simulink model "PassengerCar"  (R2019b)
settings: Solver=ode1  StartTime=0  StopTime=25  FixedStep=1.0000000000000000e-003  RelTol=1e-3
InitFcn:
  | sampleTime = str2double(get_param(bdroot, 'FixedStep'));
undefined symbols (not defined in the file or in its folder): AccPedalPos, BrakePedalPos, BrakeSwitch, DiscIntNeverNeededParam, DYNA4, EngSpd, IgnitionSwitch, InitialGear, InitialSpeed, IntendedEngTrq, LeftIndicator, MainBrakePress, MaxGear, MDL, MinGear, RefAcc, RefLane, RefLatPos, RefPath, RefPathCurv, RefSpd, RefSpdPreview, RefSpdRetrospect, RightIndicator, SteeringWheelAng, SteeringWheelTrq, UserDefinedRefValue, vm_const
libraries: UtilitiesLibrary x31, simulink x18, WheelSystemModules x13, LongitudinalControllerModules x13, LateralControllerModules x7, AnimationBusselectorModules x5, EnvironmentModules x5, BasicEngineControlModules x5, MiscellaneousControlModules x5, Animation3Modules x4, AuxiliariesModules x4, TireModules x4
(part 25 of 39)

== system PassengerCar/Vehicle/WheelSystem/RearLeftWheelSystem/WheelOutput ==
  DriveBrakeTrq_wrt_WheelRotAxis(VehSys)[Nm]___UNIQUE_1 : Inport  Description=|  PortDimensions=[3]
      | <name>DriveBrakeTrq_wrt_WheelRotAxis(VehSys)[Nm]</name>
      | <comment></comment>
  RotSpd[rad/s]___UNIQUE_1 : Inport  Description=|  Port=2  PortDimensions=[1]
      | <name>RotSpd[rad/s]</name>
      | <comment></comment>
  RotAcc[rad/s**2]___UNIQUE_1 : Inport  Description=|  Port=3  PortDimensions=[1]
      | <name>RotAcc[rad/s**2]</name>
      | <comment></comment>
  BlockingState[0;1]___UNIQUE_1 : Inport  Description=|  Port=4  PortDimensions=[1]
      | <name>BlockingState[0;1]</name>
      | <comment></comment>
  RotAng[rad]___UNIQUE_1 : Inport  Description=|  Port=5  PortDimensions=[1]
      | <name>RotAng[rad]</name>
      | <comment></comment>
  BrakeTrqPressRatio[m**3]___UNIQUE_1 : Inport  Description=|  Port=6  PortDimensions=[1]
      | <name>BrakeTrqPressRatio[m**3]</name>
      | <comment></comment>
  RotAxisInrt[kg*m**2]___UNIQUE_1 : Inport  Description=|  Port=7  PortDimensions=[1]
      | <name>RotAxisInrt[kg*m**2]</name>
      | <comment></comment>
  TotalResistanceTorque[Nm]___UNIQUE_1 : Inport  Description=|  Port=8  PortDimensions=[1]
      | <name>TotalResistanceTorque[Nm]</name>
      | <comment></comment>
  KinematicWheelActiveFlag[0;1]___UNIQUE_1 : Inport  Description=|  Port=9  PortDimensions=[1]
      | <name>KinematicWheelActiveFlag[0;1]</name>
      | <comment></comment>
  VehBodyReplacementInrt[kg*m**2]___UNIQUE_1 : Inport  Description=|  Port=10  PortDimensions=[1]
      | <name>VehBodyReplacementInrt[kg*m**2]</name>
      | <comment></comment>
  __TDD__Wheel.BlockingState[0;1] : Demux  Outputs=[1]
  __TDD__Wheel.BrakeTrqPressRatio[m**3] : Demux  Outputs=[1]
  __TDD__Wheel.DriveBrakeTrq_wrt_WheelRotAxis(VehSys)[Nm] : Demux  Outputs=[3]
  __TDD__Wheel.KinematicWheelActiveFlag[0;1] : Demux  Outputs=[1]
  __TDD__Wheel.RotAcc[rad/s**2] : Demux  Outputs=[1]
  __TDD__Wheel.RotAng[rad] : Demux  Outputs=[1]
  __TDD__Wheel.RotAxisInrt[kg*m**2] : Demux  Outputs=[1]
  __TDD__Wheel.RotSpd[rad/s] : Demux  Outputs=[1]
  __TDD__Wheel.TotalResistanceTorque[Nm] : Demux  Outputs=[1]
  __TDD__Wheel.VehBodyReplacementInrt[kg*m**2] : Demux  Outputs=[1]
  __TDO__Wheel : BusCreator  Inputs=10
  Wheel___UNIQUE_1 : Outport  Description=|  PortDimensions=[12]  VectorParamsAs1DForOutWhenUnconnected=off
      | <name>DriveBrakeTrq_wrt_WheelRotAxis(VehSys)[Nm]</name>
      | <comment></comment>
  wires:
  DriveBrakeTrq_wrt_WheelRotAxis(VehSys)[Nm]___UNIQUE_1/1 -> __TDD__Wheel.DriveBrakeTrq_wrt_WheelRotAxis(VehSys)[Nm]/1
  __TDD__Wheel.DriveBrakeTrq_wrt_WheelRotAxis(VehSys)[Nm]/1 -> __TDO__Wheel/1  "DriveBrakeTrq_wrt_WheelRotAxis(VehSys)[Nm]"
  RotSpd[rad/s]___UNIQUE_1/1 -> __TDD__Wheel.RotSpd[rad/s]/1
  __TDD__Wheel.RotSpd[rad/s]/1 -> __TDO__Wheel/2  "RotSpd[rad/s]"
  RotAcc[rad/s**2]___UNIQUE_1/1 -> __TDD__Wheel.RotAcc[rad/s**2]/1
  __TDD__Wheel.RotAcc[rad/s**2]/1 -> __TDO__Wheel/3  "RotAcc[rad/s**2]"
  BlockingState[0;1]___UNIQUE_1/1 -> __TDD__Wheel.BlockingState[0;1]/1
  __TDD__Wheel.BlockingState[0;1]/1 -> __TDO__Wheel/4  "BlockingState[0;1]"
  RotAng[rad]___UNIQUE_1/1 -> __TDD__Wheel.RotAng[rad]/1
  __TDD__Wheel.RotAng[rad]/1 -> __TDO__Wheel/5  "RotAng[rad]"
  BrakeTrqPressRatio[m**3]___UNIQUE_1/1 -> __TDD__Wheel.BrakeTrqPressRatio[m**3]/1
  __TDD__Wheel.BrakeTrqPressRatio[m**3]/1 -> __TDO__Wheel/6  "BrakeTrqPressRatio[m**3]"
  RotAxisInrt[kg*m**2]___UNIQUE_1/1 -> __TDD__Wheel.RotAxisInrt[kg*m**2]/1
  __TDD__Wheel.RotAxisInrt[kg*m**2]/1 -> __TDO__Wheel/7  "RotAxisInrt[kg*m**2]"
  TotalResistanceTorque[Nm]___UNIQUE_1/1 -> __TDD__Wheel.TotalResistanceTorque[Nm]/1
  __TDD__Wheel.TotalResistanceTorque[Nm]/1 -> __TDO__Wheel/8  "TotalResistanceTorque[Nm]"
  KinematicWheelActiveFlag[0;1]___UNIQUE_1/1 -> __TDD__Wheel.KinematicWheelActiveFlag[0;1]/1
  __TDD__Wheel.KinematicWheelActiveFlag[0;1]/1 -> __TDO__Wheel/9  "KinematicWheelActiveFlag[0;1]"
  VehBodyReplacementInrt[kg*m**2]___UNIQUE_1/1 -> __TDD__Wheel.VehBodyReplacementInrt[kg*m**2]/1
  __TDD__Wheel.VehBodyReplacementInrt[kg*m**2]/1 -> __TDO__Wheel/10  "VehBodyReplacementInrt[kg*m**2]"
  __TDO__Wheel/1 -> Wheel___UNIQUE_1/1  "Wheel"

== system PassengerCar/Vehicle/WheelSystem/RearRightWheelSystem/DynaSystemInfo ==

== system PassengerCar/Vehicle/WheelSystem/RearRightWheelSystem/InnerTireOutput ==
  __SEL__Tire.ContactPointFrc(ContactSys)[N] : Selector  InputPortWidth=1  IndexOptions=Index vector (dialog)  Indices=ones(3, 1)  OutputSizes=1
  __SEL__Tire.ContactPointPos(WorldSys)[m] : Selector  InputPortWidth=1  IndexOptions=Index vector (dialog)  Indices=ones(3, 1)  OutputSizes=1
  __SEL__Tire.ContactPointPos_wrt_WheelCenter(WorldSys)[m] : Selector  InputPortWidth=1  IndexOptions=Index vector (dialog)  Indices=ones(3, 1)  OutputSizes=1
  __SEL__Tire.LatUnitVector(WorldSys)[-] : Selector  InputPortWidth=1  IndexOptions=Index vector (dialog)  Indices=ones(3, 1)  OutputSizes=1
  __SEL__Tire.LongUnitVector(WorldSys)[-] : Selector  InputPortWidth=1  IndexOptions=Index vector (dialog)  Indices=ones(3, 1)  OutputSizes=1
  __SEL__Tire.RoadNormalVector(WorldSys)[-] : Selector  InputPortWidth=1  IndexOptions=Index vector (dialog)  Indices=ones(3, 1)  OutputSizes=1
  __SEL__Tire.WheelCenterFrc(VehSys)[N] : Selector  InputPortWidth=1  IndexOptions=Index vector (dialog)  Indices=ones(3, 1)  OutputSizes=1
  __SEL__Tire.WheelCenterTrq(VehSys)[Nm] : Selector  InputPortWidth=1  IndexOptions=Index vector (dialog)  Indices=ones(3, 1)  OutputSizes=1
  __SRC__Tire.BoreSpd(ContactSys)[rad/s] : Constant  Value=0.0  OutDataTypeStr=Inherit: Inherit via back propagation
  __SRC__Tire.CamberAng(ContactSys)[rad] : Constant  Value=0.0  OutDataTypeStr=Inherit: Inherit via back propagation
  __SRC__Tire.CircumferentialTrq_wrt_WheelRotAxis[Nm] : Constant  Value=0.0  OutDataTypeStr=Inherit: Inherit via back propagation
  __SRC__Tire.ContactPointFrc(ContactSys)[N] : Constant  Value=0.0  OutDataTypeStr=Inherit: Inherit via back propagation
  __SRC__Tire.ContactPointPos(WorldSys)[m] : Constant  Value=0.0  OutDataTypeStr=Inherit: Inherit via back propagation
  __SRC__Tire.ContactPointPos_wrt_WheelCenter(WorldSys)[m] : Constant  Value=0.0  OutDataTypeStr=Inherit: Inherit via back propagation
  __SRC__Tire.CorneringStiff[N] : Constant  Value=0.0  OutDataTypeStr=Inherit: Inherit via back propagation
  __SRC__Tire.DynamicRadius[m] : Constant  Value=0.0  OutDataTypeStr=Inherit: Inherit via back propagation
  __SRC__Tire.LatDefl(ContactSys)[m] : Constant  Value=0.0  OutDataTypeStr=Inherit: Inherit via back propagation
  __SRC__Tire.LatSpd(ContactSys)[m/s] : Constant  Value=0.0  OutDataTypeStr=Inherit: Inherit via back propagation
  __SRC__Tire.LatUnitVector(WorldSys)[-] : Constant  Value=0.0  OutDataTypeStr=Inherit: Inherit via back propagation
  __SRC__Tire.LongFrcLeverArm_wrt_WheelRotAxis[m] : Constant  Value=0.0  OutDataTypeStr=Inherit: Inherit via back propagation
  __SRC__Tire.LongSpd(ContactSys)[m/s] : Constant  Value=0.0  OutDataTypeStr=Inherit: Inherit via back propagation
  __SRC__Tire.LongUnitVector(WorldSys)[-] : Constant  Value=0.0  OutDataTypeStr=Inherit: Inherit via back propagation
  __SRC__Tire.MaxRollResistTrq[Nm] : Constant  Value=0.0  OutDataTypeStr=Inherit: Inherit via back propagation
  __SRC__Tire.RimRadius[m] : Constant  Value=0.0  OutDataTypeStr=Inherit: Inherit via back propagation
  __SRC__Tire.RoadFrictionScalingCoeff[-] : Constant  Value=0.0  OutDataTypeStr=Inherit: Inherit via back propagation
  __SRC__Tire.RoadIncl(WorldSys)[-] : Constant  Value=0.0  OutDataTypeStr=Inherit: Inherit via back propagation
  __SRC__Tire.RoadNormalVector(WorldSys)[-] : Constant  Value=0.0  OutDataTypeStr=Inherit: Inherit via back propagation
  __SRC__Tire.RoadSlope(WorldSys)[-] : Constant  Value=0.0  OutDataTypeStr=Inherit: Inherit via back propagation
  __SRC__Tire.RoadType[-] : Constant  Value=0.0  OutDataTypeStr=Inherit: Inherit via back propagation
  __SRC__Tire.Stabilization.DerivativeOfBoreTrq_wrt_BoreSpd(ContactSys)[Nm/(rad/s)] : Constant  Value=0.0  OutDataTypeStr=Inherit: Inherit via back propagation
  __SRC__Tire.Stabilization.DerivativeOfLatFrc_wrt_LatSpd(ContactSys)[N/(m/s)] : Constant  Value=0.0  OutDataTypeStr=Inherit: Inherit via back propagation
  __SRC__Tire.Stabilization.DerivativeOfLatTrq_wrt_LatSpd(ContactSys)[Nm/(m/s)] : Constant  Value=0.0  OutDataTypeStr=Inherit: Inherit via back propagation
  __SRC__Tire.Stabilization.DerivativeOfLongFrc_wrt_LongSpd(ContactSys)[N/(m/s)] : Constant  Value=0.0  OutDataTypeStr=Inherit: Inherit via back propagation
  __SRC__Tire.Stabilization.DerivativeOfLongTrq_wrt_LongSpd(ContactSys)[Nm/(m/s)] : Constant  Value=0.0  OutDataTypeStr=Inherit: Inherit via back propagation
  __SRC__Tire.TireDeflSpd[m/s] : Constant  Value=0.0  OutDataTypeStr=Inherit: Inherit via back propagation
  __SRC__Tire.TireDefl[m] : Constant  Value=0.0  OutDataTypeStr=Inherit: Inherit via back propagation
  __SRC__Tire.UnloadedRadius[m] : Constant  Value=0.0  OutDataTypeStr=Inherit: Inherit via back propagation
  __SRC__Tire.VertStiff[N/m] : Constant  Value=0.0  OutDataTypeStr=Inherit: Inherit via back propagation
  __SRC__Tire.WheelCenterFrc(VehSys)[N] : Constant  Value=0.0  OutDataTypeStr=Inherit: Inherit via back propagation
  __SRC__Tire.WheelCenterTrq(VehSys)[Nm] : Constant  Value=0.0  OutDataTypeStr=Inherit: Inherit via back propagation
  __SRC__Tire.Width[m] : Constant  Value=0.0  OutDataTypeStr=Inherit: Inherit via back propagation
  __TDO__Tire : BusCreator  Inputs=29
  __TDO__Tire.Stabilization : BusCreator  Inputs=5
  Tire___UNIQUE_1 : Outport  Description=|  PortDimensions=[49]  VectorParamsAs1DForOutWhenUnconnected=off
      | <name></name>
      | <comment></comment>
  wires:
  __SRC__Tire.ContactPointPos_wrt_WheelCenter(WorldSys)[m]/1 -> __SEL__Tire.ContactPointPos_wrt_WheelCenter(WorldSys)[m]/1
  __SRC__Tire.LongUnitVector(WorldSys)[-]/1 -> __SEL__Tire.LongUnitVector(WorldSys)[-]/1
  __SRC__Tire.LatUnitVector(WorldSys)[-]/1 -> __SEL__Tire.LatUnitVector(WorldSys)[-]/1
  __SRC__Tire.RoadNormalVector(WorldSys)[-]/1 -> __SEL__Tire.RoadNormalVector(WorldSys)[-]/1
  __SRC__Tire.ContactPointPos(WorldSys)[m]/1 -> __SEL__Tire.ContactPointPos(WorldSys)[m]/1
  __SRC__Tire.WheelCenterFrc(VehSys)[N]/1 -> __SEL__Tire.WheelCenterFrc(VehSys)[N]/1
  __SRC__Tire.WheelCenterTrq(VehSys)[Nm]/1 -> __SEL__Tire.WheelCenterTrq(VehSys)[Nm]/1
  __SRC__Tire.ContactPointFrc(ContactSys)[N]/1 -> __SEL__Tire.ContactPointFrc(ContactSys)[N]/1
  __SEL__Tire.ContactPointPos_wrt_WheelCenter(WorldSys)[m]/1 -> __TDO__Tire/1  "ContactPointPos_wrt_WheelCenter(WorldSys)[m]"
  __SRC__Tire.CamberAng(ContactSys)[rad]/1 -> __TDO__Tire/2  "CamberAng(ContactSys)[rad]"
  __SRC__Tire.TireDefl[m]/1 -> __TDO__Tire/3  "TireDefl[m]"
  __SRC__Tire.TireDeflSpd[m/s]/1 -> __TDO__Tire/4  "TireDeflSpd[m/s]"
  __SRC__Tire.LongSpd(ContactSys)[m/s]/1 -> __TDO__Tire/5  "LongSpd(ContactSys)[m/s]"
  __SRC__Tire.LatSpd(ContactSys)[m/s]/1 -> __TDO__Tire/6  "LatSpd(ContactSys)[m/s]"
  __SRC__Tire.BoreSpd(ContactSys)[rad/s]/1 -> __TDO__Tire/7  "BoreSpd(ContactSys)[rad/s]"
  __SRC__Tire.LongFrcLeverArm_wrt_WheelRotAxis[m]/1 -> __TDO__Tire/8  "LongFrcLeverArm_wrt_WheelRotAxis[m]"
  __SEL__Tire.LongUnitVector(WorldSys)[-]/1 -> __TDO__Tire/9  "LongUnitVector(WorldSys)[-]"
  __SEL__Tire.LatUnitVector(WorldSys)[-]/1 -> __TDO__Tire/10  "LatUnitVector(WorldSys)[-]"
  __SEL__Tire.RoadNormalVector(WorldSys)[-]/1 -> __TDO__Tire/11  "RoadNormalVector(WorldSys)[-]"
  __SRC__Tire.RoadType[-]/1 -> __TDO__Tire/12  "RoadType[-]"
  __SRC__Tire.RoadFrictionScalingCoeff[-]/1 -> __TDO__Tire/13  "RoadFrictionScalingCoeff[-]"
  __SEL__Tire.ContactPointPos(WorldSys)[m]/1 -> __TDO__Tire/14  "ContactPointPos(WorldSys)[m]"
  __SRC__Tire.RoadSlope(WorldSys)[-]/1 -> __TDO__Tire/15  "RoadSlope(WorldSys)[-]"
  __SRC__Tire.RoadIncl(WorldSys)[-]/1 -> __TDO__Tire/16  "RoadIncl(WorldSys)[-]"
  __SEL__Tire.WheelCenterFrc(VehSys)[N]/1 -> __TDO__Tire/17  "WheelCenterFrc(VehSys)[N]"
  __SEL__Tire.WheelCenterTrq(VehSys)[Nm]/1 -> __TDO__Tire/18  "WheelCenterTrq(VehSys)[Nm]"
  __SRC__Tire.Stabilization.DerivativeOfLongFrc_wrt_LongSpd(ContactSys)[N/(m/s)]/1 -> __TDO__Tire.Stabilization/1  "DerivativeOfLongFrc_wrt_LongSpd(ContactSys)[N/(m/s)]"
  __TDO__Tire.Stabilization/1 -> __TDO__Tire/19  "Stabilization"
  __SRC__Tire.Stabilization.DerivativeOfLongTrq_wrt_LongSpd(ContactSys)[Nm/(m/s)]/1 -> __TDO__Tire.Stabilization/2  "DerivativeOfLongTrq_wrt_LongSpd(ContactSys)[Nm/(m/s)]"
  __SRC__Tire.Stabilization.DerivativeOfLatFrc_wrt_LatSpd(ContactSys)[N/(m/s)]/1 -> __TDO__Tire.Stabilization/3  "DerivativeOfLatFrc_wrt_LatSpd(ContactSys)[N/(m/s)]"
  __SRC__Tire.Stabilization.DerivativeOfLatTrq_wrt_LatSpd(ContactSys)[Nm/(m/s)]/1 -> __TDO__Tire.Stabilization/4  "DerivativeOfLatTrq_wrt_LatSpd(ContactSys)[Nm/(m/s)]"
  __SRC__Tire.Stabilization.DerivativeOfBoreTrq_wrt_BoreSpd(ContactSys)[Nm/(rad/s)]/1 -> __TDO__Tire.Stabilization/5  "DerivativeOfBoreTrq_wrt_BoreSpd(ContactSys)[Nm/(rad/s)]"
  __SRC__Tire.CircumferentialTrq_wrt_WheelRotAxis[Nm]/1 -> __TDO__Tire/20  "CircumferentialTrq_wrt_WheelRotAxis[Nm]"
  __SRC__Tire.MaxRollResistTrq[Nm]/1 -> __TDO__Tire/21  "MaxRollResistTrq[Nm]"
  __SRC__Tire.LatDefl(ContactSys)[m]/1 -> __TDO__Tire/22  "LatDefl(ContactSys)[m]"
  __SRC__Tire.VertStiff[N/m]/1 -> __TDO__Tire/23  "VertStiff[N/m]"
  __SRC__Tire.UnloadedRadius[m]/1 -> __TDO__Tire/24  "UnloadedRadius[m]"
  __SRC__Tire.RimRadius[m]/1 -> __TDO__Tire/25  "RimRadius[m]"
  __SRC__Tire.Width[m]/1 -> __TDO__Tire/26  "Width[m]"
  __SEL__Tire.ContactPointFrc(ContactSys)[N]/1 -> __TDO__Tire/27  "ContactPointFrc(ContactSys)[N]"
  __SRC__Tire.CorneringStiff[N]/1 -> __TDO__Tire/28  "CorneringStiff[N]"
  __SRC__Tire.DynamicRadius[m]/1 -> __TDO__Tire/29  "DynamicRadius[m]"
  __TDO__Tire/1 -> Tire___UNIQUE_1/1  "Tire"
